simulink model "BasicQuadrotorControl_interface"  (R2015a)
settings: Solver=FixedStepDiscrete  StartTime=0.0  StopTime=inf  FixedStep=.001  RelTol=1e-3
model workspace (MAT data in the model file):
  clk_freq = Simulink.Parameter
  clk_freq.Value = 1000000
  clk_freq.DataType = 'uint32'
  cs_to_clk_edge = Simulink.Parameter
  cs_to_clk_edge.Value = 10
  cs_to_clk_edge.DataType = 'uint16'
  DATA_FORMAT = 12552
  init_cmd_ADXL = [11528 11528 11528 12552 12552]
  message_length = Simulink.Parameter
  message_length.Value = 16
  message_length.DataType = 'uint16'
  OUT_X_H = 45824
  OUT_X_L = 45568
  OUT_Y_H = 46336
  OUT_Y_L = 46080
  OUT_Z_H = 46848
  OUT_Z_L = 46592
  POWER_CTRL = 11528
  read_table_ADXL = [45568 45824 46080 46336 46592 46848 32768]
  stall_time = Simulink.Parameter
  stall_time.Value = 4
  stall_time.DataType = 'uint16'
  CTRL_REG1_L3G = 8399
  init_cmd_L3G = 8399
  OUT_X_H_L3G = 43264
  OUT_X_L_L3G = 43008
  OUT_Y_H_L3G = 43776
  OUT_Y_L_L3G = 43520
  OUT_Z_H_L3G = 44288
  OUT_Z_L_L3G = 44032
  read_table_L3G = [43008 43264 43520 43776 44032 44288 36608]
  WHO_AM_I_L3G = 36608
undefined symbols (not defined in the file): AXI4, Lite
libraries: axiinterfacelib x24, simulink x6
settings Model: SimulationMode=external  CovSFcnEnable=off  Creator=bsoheili  LastModifiedBy=dlwalter
settings DataIOCC: SaveOutput=off  SaveTime=off
settings OptimizationCC: BlockReduction=off  ConditionallyExecuteInputs=off  UseDivisionForNetSlopeComputation=UseDivisionForReciprocalsOfIntegersOnly  UseFloatMulNetSlope=on  EnhancedBackFolding=on  EfficientFloat2IntCast=on  OptimizeModelRefInitCode=on  LifeSpan=1  MaxStackSize=64
settings DebuggingCC: AlgebraicLoopMsg=error  SolverPrmCheckMsg=warning  InheritedTsInSrcMsg=none  StrictBusMsg=ErrorOnBusTreatedAsVector  NonBusSignalsTreatedAsBus=error
settings HardwareCC: ProdLargestAtomicInteger=Long  ProdLargestAtomicFloat=Double  ProdEndianess=LittleEndian  ProdHWDeviceType=ARM Compatible->ARM Cortex  ProdEqTarget=off
settings RTWCC: SystemTargetFile=ert.tlc  TLCOptions=-aInlineSetEventsForThisBaseRateFcn=TLC_FALSE -aSuppressMultiTaskScheduler=TLC_FALSE  TemplateMakefile=ert_default_tmf  Description=Embedded Coder  GenerateReport=on  Toolchain=Xilinx Software Development Kit (SDK) 2013.4  IncludeHyperlinkInReport=on  LaunchReport=on  GenerateTraceInfo=on  GenerateTraceReport=on  GenerateTraceReportSl=on  GenerateTraceReportSf=on  GenerateTraceReportEml=on  GenerateCodeMetricsReport=on
settings CodeAppCC: IgnoreCustomStorageClasses=off
settings ERTTargetCC: GenerateSampleERTMain=off  ParMdlRefBuildCompliant=on  CompOptLevelCompliant=on  ConcurrentExecutionCompliant=on  CombineSignalStateStructs=on  ERTFirstTimeCompliant=on  SupportContinuousTime=off  SupportVariableSizeSignals=off  ModelStepFunctionPrototypeControlCompliant=on  CPPClassGenCompliant=on

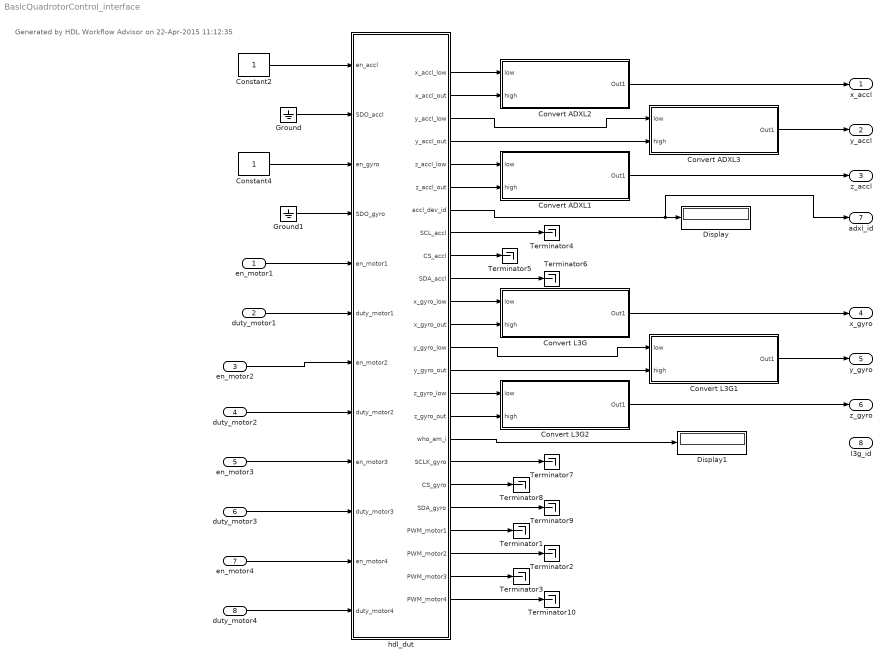
== system BasicQuadrotorControl_interface ==
  note: Generated by HDL Workflow Advisor on 22-Apr-2015 11:12:35
  en_motor1 : Inport
  duty_motor1 : Inport  Port=2
  en_motor2 : Inport  Port=3
  duty_motor2 : Inport  Port=4
  en_motor3 : Inport  Port=5
  duty_motor3 : Inport  Port=6
  en_motor4 : Inport  Port=7
  duty_motor4 : Inport  Port=8
  Constant2 : Constant  OutDataTypeStr=boolean  SampleTime=-1
  Constant4 : Constant  OutDataTypeStr=boolean  SampleTime=-1
  Convert ADXL1 : Subsystem
  Convert ADXL2 : Subsystem
  Convert ADXL3 : Subsystem
  Convert L3G : Subsystem
  Convert L3G1 : Subsystem
  Convert L3G2 : Subsystem
  Display : Display
      settings: Format=octal (Stored Integer)
  Display1 : Display
      settings: Format=binary (Stored Integer)
  Ground : Ground
  Ground1 : Ground
  Terminator{1..10} (10 alike) : Terminator
  hdl_dut : Subsystem  TreatAsAtomicUnit=on  mask(AXI4-Lite/AXI4 Interface){}
      mask help:
      | This is an automatically generated subsystem block.
      | This contains the AXI4-Lite/AXI4 interface which communicates with the BasicQuadrotorControl_hdl_dut_ipcore IPCore generated from BasicQuadrotorControl/hdl_dut subsystem.
      mask Display: disp(sprintf('Xilinx Zynq \nAXI4-Lite/AXI4 Interface'));
  x_accl : Outport
  y_accl : Outport  Port=2
  z_accl : Outport  Port=3
  x_gyro : Outport  Port=4
  y_gyro : Outport  Port=5
  z_gyro : Outport  Port=6
  adxl_id : Outport  Port=7
  l3g_id : Outport  Port=8
  wires:
  hdl_dut/21(PWM_motor1) -> Terminator1/1
  Ground1/1 -> hdl_dut/4(SDO_gyro)
  Constant4/1 -> hdl_dut/3(en_gyro)
  Constant2/1 -> hdl_dut/1(en_accl)
  Ground/1 -> hdl_dut/2(SDO_accl)
  hdl_dut/8(SCL_accl) -> Terminator4/1
  hdl_dut/9(CS_accl) -> Terminator5/1
  hdl_dut/10(SDA_accl) -> Terminator6/1
  hdl_dut/7(accl_dev_id) -> adxl_id/1, Display/1
  hdl_dut/17(who_am_i) -> Display1/1
  hdl_dut/18(SCLK_gyro) -> Terminator7/1
  hdl_dut/19(CS_gyro) -> Terminator8/1
  hdl_dut/20(SDA_gyro) -> Terminator9/1
  hdl_dut/22(PWM_motor2) -> Terminator2/1
  hdl_dut/23(PWM_motor3) -> Terminator3/1
  hdl_dut/24(PWM_motor4) -> Terminator10/1
  hdl_dut/1(x_accl_low) -> Convert ADXL2/1(low)
  hdl_dut/2(x_accl_out) -> Convert ADXL2/2(high)
  hdl_dut/5(z_accl_low) -> Convert ADXL1/1(low)
  hdl_dut/6(z_accl_out) -> Convert ADXL1/2(high)
  hdl_dut/11(x_gyro_low) -> Convert L3G/1(low)
  hdl_dut/12(x_gyro_out) -> Convert L3G/2(high)
  hdl_dut/13(y_gyro_low) -> Convert L3G1/1(low)
  hdl_dut/14(y_gyro_out) -> Convert L3G1/2(high)
  hdl_dut/15(z_gyro_low) -> Convert L3G2/1(low)
  hdl_dut/16(z_gyro_out) -> Convert L3G2/2(high)
  Convert L3G1/1(Out1) -> y_gyro/1
  Convert L3G/1(Out1) -> x_gyro/1
  Convert L3G2/1(Out1) -> z_gyro/1
  Convert ADXL1/1(Out1) -> z_accl/1
  hdl_dut/3(y_accl_low) -> Convert ADXL3/1(low)
  hdl_dut/4(y_accl_out) -> Convert ADXL3/2(high)
  Convert ADXL3/1(Out1) -> y_accl/1
  Convert ADXL2/1(Out1) -> x_accl/1
  en_motor1/1 -> hdl_dut/5(en_motor1)
  duty_motor1/1 -> hdl_dut/6(duty_motor1)
  en_motor2/1 -> hdl_dut/7(en_motor2)
  duty_motor2/1 -> hdl_dut/8(duty_motor2)
  en_motor3/1 -> hdl_dut/9(en_motor3)
  duty_motor3/1 -> hdl_dut/10(duty_motor3)
  duty_motor4/1 -> hdl_dut/12(duty_motor4)
  en_motor4/1 -> hdl_dut/11(en_motor4)
  ? -> l3g_id/1

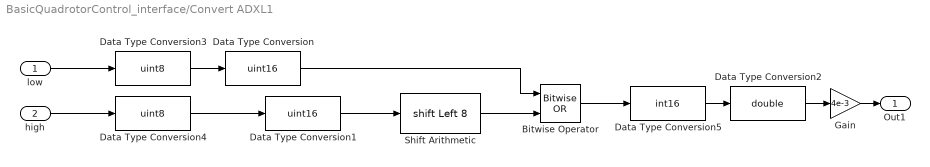
== system BasicQuadrotorControl_interface/Convert ADXL1 ==
  low : Inport
  high : Inport  Port=2
  Bitwise Operator : simulink/Logic and Bit Operations/Bitwise Operator  logicop=OR  UseBitMask=off  NumInputPorts=2  BitMask=bin2dec('11011001')  BitMaskRealWorld=Stored Integer
  Data Type Conversion : DataTypeConversion  OutDataTypeStr=uint16  ConvertRealWorld=Stored Integer (SI)
  Data Type Conversion1 : DataTypeConversion  OutDataTypeStr=uint16  ConvertRealWorld=Stored Integer (SI)
  Data Type Conversion2 : DataTypeConversion  OutDataTypeStr=double
  Data Type Conversion3 : DataTypeConversion  OutDataTypeStr=uint8
  Data Type Conversion4 : DataTypeConversion  OutDataTypeStr=uint8
  Data Type Conversion5 : DataTypeConversion  OutDataTypeStr=int16  ConvertRealWorld=Stored Integer (SI)
  Gain : Gain  Gain=4e-3
  Shift Arithmetic : ArithShift  BitShiftNumber=8  BitShiftDirection=Left
  Out1 : Outport
  wires:
  low/1 -> Data Type Conversion3/1
  Bitwise Operator/1 -> Data Type Conversion5/1
  Data Type Conversion1/1 -> Shift Arithmetic/1
  Data Type Conversion/1 -> Bitwise Operator/1
  Data Type Conversion2/1 -> Gain/1
  high/1 -> Data Type Conversion4/1
  Shift Arithmetic/1 -> Bitwise Operator/2
  Gain/1 -> Out1/1
  Data Type Conversion3/1 -> Data Type Conversion/1
  Data Type Conversion4/1 -> Data Type Conversion1/1
  Data Type Conversion5/1 -> Data Type Conversion2/1

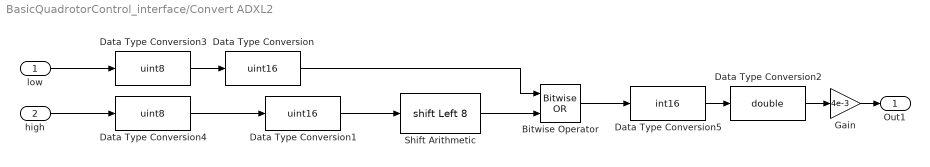
== system BasicQuadrotorControl_interface/Convert ADXL2 ==
  low : Inport
  high : Inport  Port=2
  Bitwise Operator : simulink/Logic and Bit Operations/Bitwise Operator  logicop=OR  UseBitMask=off  NumInputPorts=2  BitMask=bin2dec('11011001')  BitMaskRealWorld=Stored Integer
  Data Type Conversion : DataTypeConversion  OutDataTypeStr=uint16  ConvertRealWorld=Stored Integer (SI)
  Data Type Conversion1 : DataTypeConversion  OutDataTypeStr=uint16  ConvertRealWorld=Stored Integer (SI)
  Data Type Conversion2 : DataTypeConversion  OutDataTypeStr=double
  Data Type Conversion3 : DataTypeConversion  OutDataTypeStr=uint8
  Data Type Conversion4 : DataTypeConversion  OutDataTypeStr=uint8
  Data Type Conversion5 : DataTypeConversion  OutDataTypeStr=int16  ConvertRealWorld=Stored Integer (SI)
  Gain : Gain  Gain=4e-3
  Shift Arithmetic : ArithShift  BitShiftNumber=8  BitShiftDirection=Left
  Out1 : Outport
  wires:
  Data Type Conversion5/1 -> Data Type Conversion2/1
  Data Type Conversion4/1 -> Data Type Conversion1/1
  Data Type Conversion3/1 -> Data Type Conversion/1
  Gain/1 -> Out1/1
  Shift Arithmetic/1 -> Bitwise Operator/2
  high/1 -> Data Type Conversion4/1
  Data Type Conversion2/1 -> Gain/1
  Data Type Conversion/1 -> Bitwise Operator/1
  Data Type Conversion1/1 -> Shift Arithmetic/1
  Bitwise Operator/1 -> Data Type Conversion5/1
  low/1 -> Data Type Conversion3/1

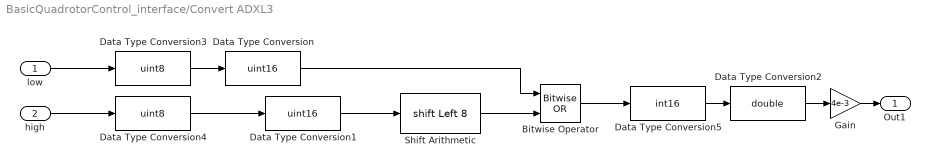
== system BasicQuadrotorControl_interface/Convert ADXL3 ==
  low : Inport
  high : Inport  Port=2
  Bitwise Operator : simulink/Logic and Bit Operations/Bitwise Operator  logicop=OR  UseBitMask=off  NumInputPorts=2  BitMask=bin2dec('11011001')  BitMaskRealWorld=Stored Integer
  Data Type Conversion : DataTypeConversion  OutDataTypeStr=uint16  ConvertRealWorld=Stored Integer (SI)
  Data Type Conversion1 : DataTypeConversion  OutDataTypeStr=uint16  ConvertRealWorld=Stored Integer (SI)
  Data Type Conversion2 : DataTypeConversion  OutDataTypeStr=double
  Data Type Conversion3 : DataTypeConversion  OutDataTypeStr=uint8
  Data Type Conversion4 : DataTypeConversion  OutDataTypeStr=uint8
  Data Type Conversion5 : DataTypeConversion  OutDataTypeStr=int16  ConvertRealWorld=Stored Integer (SI)
  Gain : Gain  Gain=4e-3
  Shift Arithmetic : ArithShift  BitShiftNumber=8  BitShiftDirection=Left
  Out1 : Outport
  wires:
  low/1 -> Data Type Conversion3/1
  Bitwise Operator/1 -> Data Type Conversion5/1
  Data Type Conversion1/1 -> Shift Arithmetic/1
  Data Type Conversion/1 -> Bitwise Operator/1
  Data Type Conversion2/1 -> Gain/1
  high/1 -> Data Type Conversion4/1
  Shift Arithmetic/1 -> Bitwise Operator/2
  Gain/1 -> Out1/1
  Data Type Conversion3/1 -> Data Type Conversion/1
  Data Type Conversion4/1 -> Data Type Conversion1/1
  Data Type Conversion5/1 -> Data Type Conversion2/1

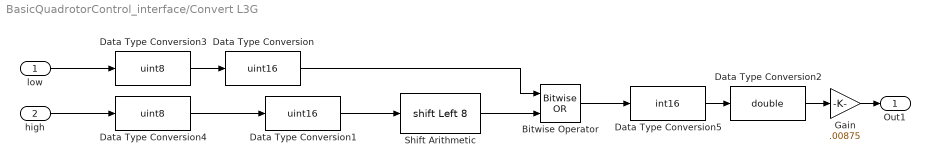
== system BasicQuadrotorControl_interface/Convert L3G ==
  low : Inport
  high : Inport  Port=2
  Bitwise Operator : simulink/Logic and Bit Operations/Bitwise Operator  logicop=OR  UseBitMask=off  NumInputPorts=2  BitMask=bin2dec('11011001')  BitMaskRealWorld=Stored Integer
  Data Type Conversion : DataTypeConversion  OutDataTypeStr=uint16  ConvertRealWorld=Stored Integer (SI)
  Data Type Conversion1 : DataTypeConversion  OutDataTypeStr=uint16  ConvertRealWorld=Stored Integer (SI)
  Data Type Conversion2 : DataTypeConversion  OutDataTypeStr=double
  Data Type Conversion3 : DataTypeConversion  OutDataTypeStr=uint8
  Data Type Conversion4 : DataTypeConversion  OutDataTypeStr=uint8
  Data Type Conversion5 : DataTypeConversion  OutDataTypeStr=int16  ConvertRealWorld=Stored Integer (SI)
  Gain : Gain  Gain=.00875
  Shift Arithmetic : ArithShift  BitShiftNumber=8  BitShiftDirection=Left
  Out1 : Outport
  wires:
  Data Type Conversion5/1 -> Data Type Conversion2/1
  Data Type Conversion4/1 -> Data Type Conversion1/1
  Data Type Conversion3/1 -> Data Type Conversion/1
  Gain/1 -> Out1/1
  Shift Arithmetic/1 -> Bitwise Operator/2
  high/1 -> Data Type Conversion4/1
  Data Type Conversion2/1 -> Gain/1
  Data Type Conversion/1 -> Bitwise Operator/1
  Data Type Conversion1/1 -> Shift Arithmetic/1
  Bitwise Operator/1 -> Data Type Conversion5/1
  low/1 -> Data Type Conversion3/1

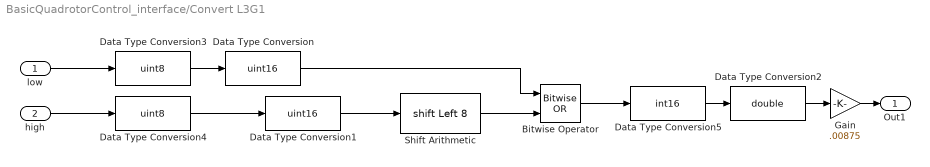
== system BasicQuadrotorControl_interface/Convert L3G1 ==
  low : Inport
  high : Inport  Port=2
  Bitwise Operator : simulink/Logic and Bit Operations/Bitwise Operator  logicop=OR  UseBitMask=off  NumInputPorts=2  BitMask=bin2dec('11011001')  BitMaskRealWorld=Stored Integer
  Data Type Conversion : DataTypeConversion  OutDataTypeStr=uint16  ConvertRealWorld=Stored Integer (SI)
  Data Type Conversion1 : DataTypeConversion  OutDataTypeStr=uint16  ConvertRealWorld=Stored Integer (SI)
  Data Type Conversion2 : DataTypeConversion  OutDataTypeStr=double
  Data Type Conversion3 : DataTypeConversion  OutDataTypeStr=uint8
  Data Type Conversion4 : DataTypeConversion  OutDataTypeStr=uint8
  Data Type Conversion5 : DataTypeConversion  OutDataTypeStr=int16  ConvertRealWorld=Stored Integer (SI)
  Gain : Gain  Gain=.00875
  Shift Arithmetic : ArithShift  BitShiftNumber=8  BitShiftDirection=Left
  Out1 : Outport
  wires:
  low/1 -> Data Type Conversion3/1
  Bitwise Operator/1 -> Data Type Conversion5/1
  Data Type Conversion1/1 -> Shift Arithmetic/1
  Data Type Conversion/1 -> Bitwise Operator/1
  Data Type Conversion2/1 -> Gain/1
  high/1 -> Data Type Conversion4/1
  Shift Arithmetic/1 -> Bitwise Operator/2
  Gain/1 -> Out1/1
  Data Type Conversion3/1 -> Data Type Conversion/1
  Data Type Conversion4/1 -> Data Type Conversion1/1
  Data Type Conversion5/1 -> Data Type Conversion2/1

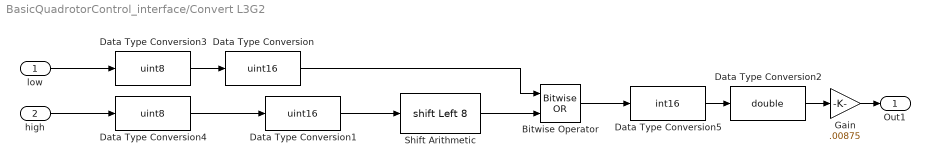
== system BasicQuadrotorControl_interface/Convert L3G2 ==
  low : Inport
  high : Inport  Port=2
  Bitwise Operator : simulink/Logic and Bit Operations/Bitwise Operator  logicop=OR  UseBitMask=off  NumInputPorts=2  BitMask=bin2dec('11011001')  BitMaskRealWorld=Stored Integer
  Data Type Conversion : DataTypeConversion  OutDataTypeStr=uint16  ConvertRealWorld=Stored Integer (SI)
  Data Type Conversion1 : DataTypeConversion  OutDataTypeStr=uint16  ConvertRealWorld=Stored Integer (SI)
  Data Type Conversion2 : DataTypeConversion  OutDataTypeStr=double
  Data Type Conversion3 : DataTypeConversion  OutDataTypeStr=uint8
  Data Type Conversion4 : DataTypeConversion  OutDataTypeStr=uint8
  Data Type Conversion5 : DataTypeConversion  OutDataTypeStr=int16  ConvertRealWorld=Stored Integer (SI)
  Gain : Gain  Gain=.00875
  Shift Arithmetic : ArithShift  BitShiftNumber=8  BitShiftDirection=Left
  Out1 : Outport
  wires:
  Data Type Conversion5/1 -> Data Type Conversion2/1
  Data Type Conversion4/1 -> Data Type Conversion1/1
  Data Type Conversion3/1 -> Data Type Conversion/1
  Gain/1 -> Out1/1
  Shift Arithmetic/1 -> Bitwise Operator/2
  high/1 -> Data Type Conversion4/1
  Data Type Conversion2/1 -> Gain/1
  Data Type Conversion/1 -> Bitwise Operator/1
  Data Type Conversion1/1 -> Shift Arithmetic/1
  Bitwise Operator/1 -> Data Type Conversion5/1
  low/1 -> Data Type Conversion3/1

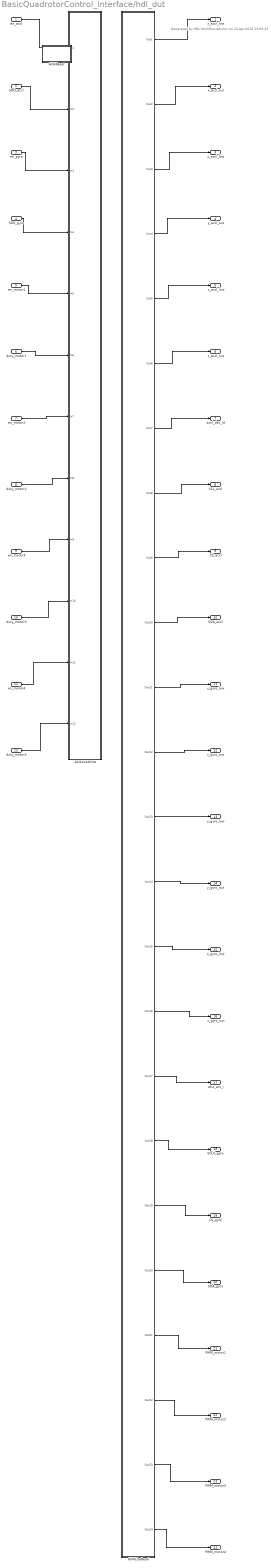
== system BasicQuadrotorControl_interface/hdl_dut ==
  note: Generated by HDL Workflow Advisor on 22-Apr-2015 13:00:23
  en_accl : Inport
  SDO_accl : Inport  Port=2
  en_gyro : Inport  Port=3
  SDO_gyro : Inport  Port=4
  en_motor1 : Inport  Port=5
  duty_motor1 : Inport  Port=6
  en_motor2 : Inport  Port=7
  duty_motor2 : Inport  Port=8
  en_motor3 : Inport  Port=9
  duty_motor3 : Inport  Port=10
  en_motor4 : Inport  Port=11
  duty_motor4 : Inport  Port=12
  AXI4LiteRead : Subsystem  Priority=10
  AXI4LiteWrite : Subsystem  Priority=1
  AXI4Reset : Subsystem  mask(System Initialize){ShowInLibBrowser=0}
      mask prompts: ShowInLibBrowser "Simulink:masks:CustCodeMaskParam1_MP"
      settings: CopyFcn=cccopyfcn(gcb)  OpenFcn=ccopenfcn('System Initialize Function')
      mask Help: eval('feval(''rtwprivate'',''rtwhelpview'',''rtw_sys_initialize_block'')');
      mask Display: disp('System\nInitialize');
  x_accl_low : Outport
  x_accl_out : Outport  Port=2
  y_accl_low : Outport  Port=3
  y_accl_out : Outport  Port=4
  z_accl_low : Outport  Port=5
  z_accl_out : Outport  Port=6
  accl_dev_id : Outport  Port=7
  SCL_accl : Outport  Port=8
  CS_accl : Outport  Port=9
  SDA_accl : Outport  Port=10
  x_gyro_low : Outport  Port=11
  x_gyro_out : Outport  Port=12
  y_gyro_low : Outport  Port=13
  y_gyro_out : Outport  Port=14
  z_gyro_low : Outport  Port=15
  z_gyro_out : Outport  Port=16
  who_am_i : Outport  Port=17
  SCLK_gyro : Outport  Port=18
  CS_gyro : Outport  Port=19
  SDA_gyro : Outport  Port=20
  PWM_motor1 : Outport  Port=21  OutDataTypeStr=boolean
  PWM_motor2 : Outport  Port=22  OutDataTypeStr=boolean
  PWM_motor3 : Outport  Port=23  OutDataTypeStr=boolean
  PWM_motor4 : Outport  Port=24  OutDataTypeStr=boolean
  wires:
  en_accl/1 -> AXI4LiteWrite/1(In1)
  SDO_accl/1 -> AXI4LiteWrite/2(In2)
  en_gyro/1 -> AXI4LiteWrite/3(In3)
  SDO_gyro/1 -> AXI4LiteWrite/4(In4)
  en_motor1/1 -> AXI4LiteWrite/5(In5)
  duty_motor1/1 -> AXI4LiteWrite/6(In6)
  en_motor2/1 -> AXI4LiteWrite/7(In7)
  duty_motor2/1 -> AXI4LiteWrite/8(In8)
  en_motor3/1 -> AXI4LiteWrite/9(In9)
  duty_motor3/1 -> AXI4LiteWrite/10(In10)
  en_motor4/1 -> AXI4LiteWrite/11(In11)
  duty_motor4/1 -> AXI4LiteWrite/12(In12)
  AXI4LiteRead/1(Out1) -> x_accl_low/1
  AXI4LiteRead/2(Out2) -> x_accl_out/1
  AXI4LiteRead/3(Out3) -> y_accl_low/1
  AXI4LiteRead/4(Out4) -> y_accl_out/1
  AXI4LiteRead/5(Out5) -> z_accl_low/1
  AXI4LiteRead/6(Out6) -> z_accl_out/1
  AXI4LiteRead/7(Out7) -> accl_dev_id/1
  AXI4LiteRead/8(Out8) -> SCL_accl/1
  AXI4LiteRead/9(Out9) -> CS_accl/1
  AXI4LiteRead/10(Out10) -> SDA_accl/1
  AXI4LiteRead/11(Out11) -> x_gyro_low/1
  AXI4LiteRead/12(Out12) -> x_gyro_out/1
  AXI4LiteRead/13(Out13) -> y_gyro_low/1
  AXI4LiteRead/14(Out14) -> y_gyro_out/1
  AXI4LiteRead/15(Out15) -> z_gyro_low/1
  AXI4LiteRead/16(Out16) -> z_gyro_out/1
  AXI4LiteRead/17(Out17) -> who_am_i/1
  AXI4LiteRead/18(Out18) -> SCLK_gyro/1
  AXI4LiteRead/19(Out19) -> CS_gyro/1
  AXI4LiteRead/20(Out20) -> SDA_gyro/1
  AXI4LiteRead/21(Out21) -> PWM_motor1/1
  AXI4LiteRead/22(Out22) -> PWM_motor2/1
  AXI4LiteRead/23(Out23) -> PWM_motor3/1
  AXI4LiteRead/24(Out24) -> PWM_motor4/1

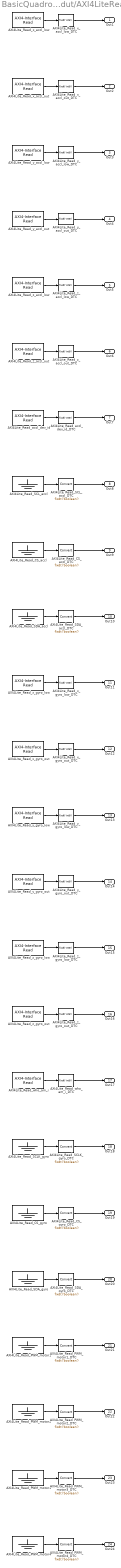
== system BasicQuadrotorControl_interface/hdl_dut/AXI4LiteRead ==
  AXI4Lite_Read_CS_accl : Ground
  AXI4Lite_Read_CS_accl_DTC : DataTypeConversion  OutDataTypeStr=fixdt('boolean')  ConvertRealWorld=Stored Integer (SI)
  AXI4Lite_Read_CS_gyro : Ground
  AXI4Lite_Read_CS_gyro_DTC : DataTypeConversion  OutDataTypeStr=fixdt('boolean')  ConvertRealWorld=Stored Integer (SI)
  AXI4Lite_Read_PWM_motor{1..4} (4 alike) : Ground
  AXI4Lite_Read_PWM_motor1_DTC : DataTypeConversion  OutDataTypeStr=fixdt('boolean')  ConvertRealWorld=Stored Integer (SI)
  AXI4Lite_Read_PWM_motor2_DTC : DataTypeConversion  OutDataTypeStr=fixdt('boolean')  ConvertRealWorld=Stored Integer (SI)
  AXI4Lite_Read_PWM_motor3_DTC : DataTypeConversion  OutDataTypeStr=fixdt('boolean')  ConvertRealWorld=Stored Integer (SI)
  AXI4Lite_Read_PWM_motor4_DTC : DataTypeConversion  OutDataTypeStr=fixdt('boolean')  ConvertRealWorld=Stored Integer (SI)
  AXI4Lite_Read_SCLK_gyro : Ground
  AXI4Lite_Read_SCLK_gyro_DTC : DataTypeConversion  OutDataTypeStr=fixdt('boolean')  ConvertRealWorld=Stored Integer (SI)
  AXI4Lite_Read_SCL_accl : Ground
  AXI4Lite_Read_SCL_accl_DTC : DataTypeConversion  OutDataTypeStr=fixdt('boolean')  ConvertRealWorld=Stored Integer (SI)
  AXI4Lite_Read_SDA_accl : Ground
  AXI4Lite_Read_SDA_accl_DTC : DataTypeConversion  OutDataTypeStr=fixdt('boolean')  ConvertRealWorld=Stored Integer (SI)
  AXI4Lite_Read_SDA_gyro : Ground
  AXI4Lite_Read_SDA_gyro_DTC : DataTypeConversion  OutDataTypeStr=fixdt('boolean')  ConvertRealWorld=Stored Integer (SI)
  AXI4Lite_Read_accl_dev_id : axiinterfacelib/AXI4-Interface Read  Priority=8  AXIInterfaceType=AXI4-Lite  DeviceName=/dev/mwipcore  RegisterOffset=hex2dec('140')  DataLength=4096  DataType=uint32  SampleTime=-1  blockPlatform=ZYNQ  SimulateUsing=Interpreted Execution
  AXI4Lite_Read_accl_dev_id_DTC : DataTypeConversion  OutDataTypeStr=fixdt('int8')  ConvertRealWorld=Stored Integer (SI)
  AXI4Lite_Read_who_am_i : axiinterfacelib/AXI4-Interface Read  Priority=18  AXIInterfaceType=AXI4-Lite  DeviceName=/dev/mwipcore  RegisterOffset=hex2dec('15C')  DataLength=4096  DataType=uint32  SampleTime=-1  blockPlatform=ZYNQ  SimulateUsing=Interpreted Execution
  AXI4Lite_Read_who_am_i_DTC : DataTypeConversion  OutDataTypeStr=fixdt('int8')  ConvertRealWorld=Stored Integer (SI)
  AXI4Lite_Read_x_accl_low : axiinterfacelib/AXI4-Interface Read  Priority=2  AXIInterfaceType=AXI4-Lite  DeviceName=/dev/mwipcore  RegisterOffset=hex2dec('128')  DataLength=4096  DataType=uint32  SampleTime=-1  blockPlatform=ZYNQ  SimulateUsing=Interpreted Execution
  AXI4Lite_Read_x_accl_low_DTC : DataTypeConversion  OutDataTypeStr=fixdt('int8')  ConvertRealWorld=Stored Integer (SI)
  AXI4Lite_Read_x_accl_out : axiinterfacelib/AXI4-Interface Read  Priority=3  AXIInterfaceType=AXI4-Lite  DeviceName=/dev/mwipcore  RegisterOffset=hex2dec('12C')  DataLength=4096  DataType=uint32  SampleTime=-1  blockPlatform=ZYNQ  SimulateUsing=Interpreted Execution
  AXI4Lite_Read_x_accl_out_DTC : DataTypeConversion  OutDataTypeStr=fixdt('int8')  ConvertRealWorld=Stored Integer (SI)
  AXI4Lite_Read_x_gyro_low : axiinterfacelib/AXI4-Interface Read  Priority=12  AXIInterfaceType=AXI4-Lite  DeviceName=/dev/mwipcore  RegisterOffset=hex2dec('144')  DataLength=4096  DataType=uint32  SampleTime=-1  blockPlatform=ZYNQ  SimulateUsing=Interpreted Execution
  AXI4Lite_Read_x_gyro_low_DTC : DataTypeConversion  OutDataTypeStr=fixdt('int8')  ConvertRealWorld=Stored Integer (SI)
  AXI4Lite_Read_x_gyro_out : axiinterfacelib/AXI4-Interface Read  Priority=13  AXIInterfaceType=AXI4-Lite  DeviceName=/dev/mwipcore  RegisterOffset=hex2dec('148')  DataLength=4096  DataType=uint32  SampleTime=-1  blockPlatform=ZYNQ  SimulateUsing=Interpreted Execution
  AXI4Lite_Read_x_gyro_out_DTC : DataTypeConversion  OutDataTypeStr=fixdt('int8')  ConvertRealWorld=Stored Integer (SI)
  AXI4Lite_Read_y_accl_low : axiinterfacelib/AXI4-Interface Read  Priority=4  AXIInterfaceType=AXI4-Lite  DeviceName=/dev/mwipcore  RegisterOffset=hex2dec('130')  DataLength=4096  DataType=uint32  SampleTime=-1  blockPlatform=ZYNQ  SimulateUsing=Interpreted Execution
  AXI4Lite_Read_y_accl_low_DTC : DataTypeConversion  OutDataTypeStr=fixdt('int8')  ConvertRealWorld=Stored Integer (SI)
  AXI4Lite_Read_y_accl_out : axiinterfacelib/AXI4-Interface Read  Priority=5  AXIInterfaceType=AXI4-Lite  DeviceName=/dev/mwipcore  RegisterOffset=hex2dec('134')  DataLength=4096  DataType=uint32  SampleTime=-1  blockPlatform=ZYNQ  SimulateUsing=Interpreted Execution
  AXI4Lite_Read_y_accl_out_DTC : DataTypeConversion  OutDataTypeStr=fixdt('int8')  ConvertRealWorld=Stored Integer (SI)
  AXI4Lite_Read_y_gyro_low : axiinterfacelib/AXI4-Interface Read  Priority=14  AXIInterfaceType=AXI4-Lite  DeviceName=/dev/mwipcore  RegisterOffset=hex2dec('14C')  DataLength=4096  DataType=uint32  SampleTime=-1  blockPlatform=ZYNQ  SimulateUsing=Interpreted Execution
  AXI4Lite_Read_y_gyro_low_DTC : DataTypeConversion  OutDataTypeStr=fixdt('int8')  ConvertRealWorld=Stored Integer (SI)
  AXI4Lite_Read_y_gyro_out : axiinterfacelib/AXI4-Interface Read  Priority=15  AXIInterfaceType=AXI4-Lite  DeviceName=/dev/mwipcore  RegisterOffset=hex2dec('150')  DataLength=4096  DataType=uint32  SampleTime=-1  blockPlatform=ZYNQ  SimulateUsing=Interpreted Execution
  AXI4Lite_Read_y_gyro_out_DTC : DataTypeConversion  OutDataTypeStr=fixdt('int8')  ConvertRealWorld=Stored Integer (SI)
  AXI4Lite_Read_z_accl_low : axiinterfacelib/AXI4-Interface Read  Priority=6  AXIInterfaceType=AXI4-Lite  DeviceName=/dev/mwipcore  RegisterOffset=hex2dec('138')  DataLength=4096  DataType=uint32  SampleTime=-1  blockPlatform=ZYNQ  SimulateUsing=Interpreted Execution
  AXI4Lite_Read_z_accl_low_DTC : DataTypeConversion  OutDataTypeStr=fixdt('int8')  ConvertRealWorld=Stored Integer (SI)
  AXI4Lite_Read_z_accl_out : axiinterfacelib/AXI4-Interface Read  Priority=7  AXIInterfaceType=AXI4-Lite  DeviceName=/dev/mwipcore  RegisterOffset=hex2dec('13C')  DataLength=4096  DataType=uint32  SampleTime=-1  blockPlatform=ZYNQ  SimulateUsing=Interpreted Execution
  AXI4Lite_Read_z_accl_out_DTC : DataTypeConversion  OutDataTypeStr=fixdt('int8')  ConvertRealWorld=Stored Integer (SI)
  AXI4Lite_Read_z_gyro_low : axiinterfacelib/AXI4-Interface Read  Priority=16  AXIInterfaceType=AXI4-Lite  DeviceName=/dev/mwipcore  RegisterOffset=hex2dec('154')  DataLength=4096  DataType=uint32  SampleTime=-1  blockPlatform=ZYNQ  SimulateUsing=Interpreted Execution
  AXI4Lite_Read_z_gyro_low_DTC : DataTypeConversion  OutDataTypeStr=fixdt('int8')  ConvertRealWorld=Stored Integer (SI)
  AXI4Lite_Read_z_gyro_out : axiinterfacelib/AXI4-Interface Read  Priority=17  AXIInterfaceType=AXI4-Lite  DeviceName=/dev/mwipcore  RegisterOffset=hex2dec('158')  DataLength=4096  DataType=uint32  SampleTime=-1  blockPlatform=ZYNQ  SimulateUsing=Interpreted Execution
  AXI4Lite_Read_z_gyro_out_DTC : DataTypeConversion  OutDataTypeStr=fixdt('int8')  ConvertRealWorld=Stored Integer (SI)
  Out1 : Outport
  Out2 : Outport  Port=2
  Out3 : Outport  Port=3
  Out4 : Outport  Port=4
  Out5 : Outport  Port=5
  Out6 : Outport  Port=6
  Out7 : Outport  Port=7
  Out8 : Outport  Port=8
  Out9 : Outport  Port=9
  Out10 : Outport  Port=10
  Out11 : Outport  Port=11
  Out12 : Outport  Port=12
  Out13 : Outport  Port=13
  Out14 : Outport  Port=14
  Out15 : Outport  Port=15
  Out16 : Outport  Port=16
  Out17 : Outport  Port=17
  Out18 : Outport  Port=18
  Out19 : Outport  Port=19
  Out20 : Outport  Port=20
  Out21 : Outport  Port=21
  Out22 : Outport  Port=22
  Out23 : Outport  Port=23
  Out24 : Outport  Port=24
  wires:
  AXI4Lite_Read_SCL_accl/1 -> AXI4Lite_Read_SCL_accl_DTC/1
  AXI4Lite_Read_SCL_accl_DTC/1 -> Out8/1
  AXI4Lite_Read_accl_dev_id_DTC/1 -> Out7/1
  AXI4Lite_Read_accl_dev_id/1 -> AXI4Lite_Read_accl_dev_id_DTC/1
  AXI4Lite_Read_CS_accl/1 -> AXI4Lite_Read_CS_accl_DTC/1
  AXI4Lite_Read_CS_accl_DTC/1 -> Out9/1
  AXI4Lite_Read_SDA_accl/1 -> AXI4Lite_Read_SDA_accl_DTC/1
  AXI4Lite_Read_SDA_accl_DTC/1 -> Out10/1
  AXI4Lite_Read_x_gyro_low/1 -> AXI4Lite_Read_x_gyro_low_DTC/1
  AXI4Lite_Read_x_gyro_low_DTC/1 -> Out11/1
  AXI4Lite_Read_y_gyro_low_DTC/1 -> Out13/1
  AXI4Lite_Read_y_gyro_low/1 -> AXI4Lite_Read_y_gyro_low_DTC/1
  AXI4Lite_Read_y_gyro_out/1 -> AXI4Lite_Read_y_gyro_out_DTC/1
  AXI4Lite_Read_y_gyro_out_DTC/1 -> Out14/1
  AXI4Lite_Read_z_gyro_low_DTC/1 -> Out15/1
  AXI4Lite_Read_z_gyro_low/1 -> AXI4Lite_Read_z_gyro_low_DTC/1
  AXI4Lite_Read_z_gyro_out_DTC/1 -> Out16/1
  AXI4Lite_Read_z_gyro_out/1 -> AXI4Lite_Read_z_gyro_out_DTC/1
  AXI4Lite_Read_who_am_i_DTC/1 -> Out17/1
  AXI4Lite_Read_SCLK_gyro/1 -> AXI4Lite_Read_SCLK_gyro_DTC/1
  AXI4Lite_Read_who_am_i/1 -> AXI4Lite_Read_who_am_i_DTC/1
  AXI4Lite_Read_SCLK_gyro_DTC/1 -> Out18/1
  AXI4Lite_Read_CS_gyro/1 -> AXI4Lite_Read_CS_gyro_DTC/1
  AXI4Lite_Read_SDA_gyro_DTC/1 -> Out20/1
  AXI4Lite_Read_PWM_motor1/1 -> AXI4Lite_Read_PWM_motor1_DTC/1
  AXI4Lite_Read_PWM_motor3_DTC/1 -> Out23/1
  AXI4Lite_Read_PWM_motor4/1 -> AXI4Lite_Read_PWM_motor4_DTC/1
  AXI4Lite_Read_PWM_motor2_DTC/1 -> Out22/1
  AXI4Lite_Read_PWM_motor2/1 -> AXI4Lite_Read_PWM_motor2_DTC/1
  AXI4Lite_Read_PWM_motor1_DTC/1 -> Out21/1
  AXI4Lite_Read_PWM_motor3/1 -> AXI4Lite_Read_PWM_motor3_DTC/1
  AXI4Lite_Read_CS_gyro_DTC/1 -> Out19/1
  AXI4Lite_Read_SDA_gyro/1 -> AXI4Lite_Read_SDA_gyro_DTC/1
  AXI4Lite_Read_PWM_motor4_DTC/1 -> Out24/1
  AXI4Lite_Read_x_gyro_out/1 -> AXI4Lite_Read_x_gyro_out_DTC/1
  AXI4Lite_Read_x_gyro_out_DTC/1 -> Out12/1
  AXI4Lite_Read_z_accl_low_DTC/1 -> Out5/1
  AXI4Lite_Read_z_accl_low/1 -> AXI4Lite_Read_z_accl_low_DTC/1
  AXI4Lite_Read_z_accl_out/1 -> AXI4Lite_Read_z_accl_out_DTC/1
  AXI4Lite_Read_z_accl_out_DTC/1 -> Out6/1
  AXI4Lite_Read_x_accl_out/1 -> AXI4Lite_Read_x_accl_out_DTC/1
  AXI4Lite_Read_x_accl_out_DTC/1 -> Out2/1
  AXI4Lite_Read_y_accl_low/1 -> AXI4Lite_Read_y_accl_low_DTC/1
  AXI4Lite_Read_y_accl_low_DTC/1 -> Out3/1
  AXI4Lite_Read_y_accl_out/1 -> AXI4Lite_Read_y_accl_out_DTC/1
  AXI4Lite_Read_x_accl_low/1 -> AXI4Lite_Read_x_accl_low_DTC/1
  AXI4Lite_Read_x_accl_low_DTC/1 -> Out1/1
  AXI4Lite_Read_y_accl_out_DTC/1 -> Out4/1

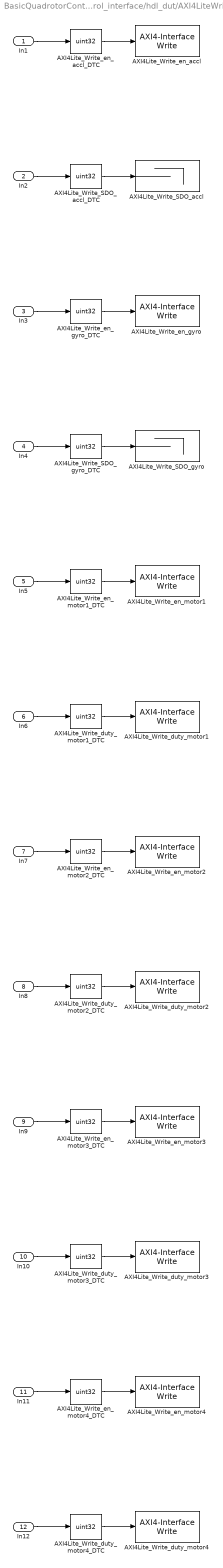
== system BasicQuadrotorControl_interface/hdl_dut/AXI4LiteWrite ==
  In1 : Inport
  In2 : Inport  Port=2
  In3 : Inport  Port=3
  In4 : Inport  Port=4
  In5 : Inport  Port=5
  In6 : Inport  Port=6
  In7 : Inport  Port=7
  In8 : Inport  Port=8
  In9 : Inport  Port=9
  In10 : Inport  Port=10
  In11 : Inport  Port=11
  In12 : Inport  Port=12
  AXI4Lite_Write_SDO_accl : Terminator
  AXI4Lite_Write_SDO_accl_DTC : DataTypeConversion  OutDataTypeStr=uint32  ConvertRealWorld=Stored Integer (SI)
  AXI4Lite_Write_SDO_gyro : Terminator
  AXI4Lite_Write_SDO_gyro_DTC : DataTypeConversion  OutDataTypeStr=uint32  ConvertRealWorld=Stored Integer (SI)
  AXI4Lite_Write_duty_motor1 : axiinterfacelib/AXI4-Interface Write  Priority=6  AXIInterfaceType=AXI4-Lite  DeviceName=/dev/mwipcore  RegisterOffset=hex2dec('10C')  blockPlatform=ZYNQ  SimulateUsing=Interpreted execution
  AXI4Lite_Write_duty_motor1_DTC : DataTypeConversion  OutDataTypeStr=uint32  ConvertRealWorld=Stored Integer (SI)
  AXI4Lite_Write_duty_motor2 : axiinterfacelib/AXI4-Interface Write  Priority=8  AXIInterfaceType=AXI4-Lite  DeviceName=/dev/mwipcore  RegisterOffset=hex2dec('114')  blockPlatform=ZYNQ  SimulateUsing=Interpreted execution
  AXI4Lite_Write_duty_motor2_DTC : DataTypeConversion  OutDataTypeStr=uint32  ConvertRealWorld=Stored Integer (SI)
  AXI4Lite_Write_duty_motor3 : axiinterfacelib/AXI4-Interface Write  Priority=10  AXIInterfaceType=AXI4-Lite  DeviceName=/dev/mwipcore  RegisterOffset=hex2dec('11C')  blockPlatform=ZYNQ  SimulateUsing=Interpreted execution
  AXI4Lite_Write_duty_motor3_DTC : DataTypeConversion  OutDataTypeStr=uint32  ConvertRealWorld=Stored Integer (SI)
  AXI4Lite_Write_duty_motor4 : axiinterfacelib/AXI4-Interface Write  Priority=12  AXIInterfaceType=AXI4-Lite  DeviceName=/dev/mwipcore  RegisterOffset=hex2dec('124')  blockPlatform=ZYNQ  SimulateUsing=Interpreted execution
  AXI4Lite_Write_duty_motor4_DTC : DataTypeConversion  OutDataTypeStr=uint32  ConvertRealWorld=Stored Integer (SI)
  AXI4Lite_Write_en_accl : axiinterfacelib/AXI4-Interface Write  Priority=1  AXIInterfaceType=AXI4-Lite  DeviceName=/dev/mwipcore  RegisterOffset=hex2dec('100')  blockPlatform=ZYNQ  SimulateUsing=Interpreted execution
  AXI4Lite_Write_en_accl_DTC : DataTypeConversion  OutDataTypeStr=uint32  ConvertRealWorld=Stored Integer (SI)
  AXI4Lite_Write_en_gyro : axiinterfacelib/AXI4-Interface Write  Priority=3  AXIInterfaceType=AXI4-Lite  DeviceName=/dev/mwipcore  RegisterOffset=hex2dec('104')  blockPlatform=ZYNQ  SimulateUsing=Interpreted execution
  AXI4Lite_Write_en_gyro_DTC : DataTypeConversion  OutDataTypeStr=uint32  ConvertRealWorld=Stored Integer (SI)
  AXI4Lite_Write_en_motor1 : axiinterfacelib/AXI4-Interface Write  Priority=5  AXIInterfaceType=AXI4-Lite  DeviceName=/dev/mwipcore  RegisterOffset=hex2dec('108')  blockPlatform=ZYNQ  SimulateUsing=Interpreted execution
  AXI4Lite_Write_en_motor1_DTC : DataTypeConversion  OutDataTypeStr=uint32  ConvertRealWorld=Stored Integer (SI)
  AXI4Lite_Write_en_motor2 : axiinterfacelib/AXI4-Interface Write  Priority=7  AXIInterfaceType=AXI4-Lite  DeviceName=/dev/mwipcore  RegisterOffset=hex2dec('110')  blockPlatform=ZYNQ  SimulateUsing=Interpreted execution
  AXI4Lite_Write_en_motor2_DTC : DataTypeConversion  OutDataTypeStr=uint32  ConvertRealWorld=Stored Integer (SI)
  AXI4Lite_Write_en_motor3 : axiinterfacelib/AXI4-Interface Write  Priority=9  AXIInterfaceType=AXI4-Lite  DeviceName=/dev/mwipcore  RegisterOffset=hex2dec('118')  blockPlatform=ZYNQ  SimulateUsing=Interpreted execution
  AXI4Lite_Write_en_motor3_DTC : DataTypeConversion  OutDataTypeStr=uint32  ConvertRealWorld=Stored Integer (SI)
  AXI4Lite_Write_en_motor4 : axiinterfacelib/AXI4-Interface Write  Priority=11  AXIInterfaceType=AXI4-Lite  DeviceName=/dev/mwipcore  RegisterOffset=hex2dec('120')  blockPlatform=ZYNQ  SimulateUsing=Interpreted execution
  AXI4Lite_Write_en_motor4_DTC : DataTypeConversion  OutDataTypeStr=uint32  ConvertRealWorld=Stored Integer (SI)
  wires:
  In8/1 -> AXI4Lite_Write_duty_motor2_DTC/1
  AXI4Lite_Write_duty_motor4_DTC/1 -> AXI4Lite_Write_duty_motor4/1
  In12/1 -> AXI4Lite_Write_duty_motor4_DTC/1
  AXI4Lite_Write_duty_motor2_DTC/1 -> AXI4Lite_Write_duty_motor2/1
  In9/1 -> AXI4Lite_Write_en_motor3_DTC/1
  AXI4Lite_Write_en_motor3_DTC/1 -> AXI4Lite_Write_en_motor3/1
  AXI4Lite_Write_en_motor4_DTC/1 -> AXI4Lite_Write_en_motor4/1
  In10/1 -> AXI4Lite_Write_duty_motor3_DTC/1
  In11/1 -> AXI4Lite_Write_en_motor4_DTC/1
  AXI4Lite_Write_duty_motor3_DTC/1 -> AXI4Lite_Write_duty_motor3/1
  AXI4Lite_Write_en_motor2_DTC/1 -> AXI4Lite_Write_en_motor2/1
  In3/1 -> AXI4Lite_Write_en_gyro_DTC/1
  AXI4Lite_Write_en_gyro_DTC/1 -> AXI4Lite_Write_en_gyro/1
  In4/1 -> AXI4Lite_Write_SDO_gyro_DTC/1
  AXI4Lite_Write_SDO_gyro_DTC/1 -> AXI4Lite_Write_SDO_gyro/1
  AXI4Lite_Write_en_motor1_DTC/1 -> AXI4Lite_Write_en_motor1/1
  In5/1 -> AXI4Lite_Write_en_motor1_DTC/1
  In6/1 -> AXI4Lite_Write_duty_motor1_DTC/1
  AXI4Lite_Write_duty_motor1_DTC/1 -> AXI4Lite_Write_duty_motor1/1
  AXI4Lite_Write_SDO_accl_DTC/1 -> AXI4Lite_Write_SDO_accl/1
  AXI4Lite_Write_en_accl_DTC/1 -> AXI4Lite_Write_en_accl/1
  In1/1 -> AXI4Lite_Write_en_accl_DTC/1
  In2/1 -> AXI4Lite_Write_SDO_accl_DTC/1
  In7/1 -> AXI4Lite_Write_en_motor2_DTC/1

== system BasicQuadrotorControl_interface/hdl_dut/AXI4Reset ==
